simulink model "LAB_BalancingRobotSim"  (R2020b)
settings: Solver=FixedStepDiscrete  StartTime=0.0  StopTime=10.0  FixedStep=0.01  RelTol=1e-3  EnableMultiTasking=on
undefined symbols (not defined in the file): D_CF, DiscIntNeverNeededParam, drv, gbox, H, K, K_I, Ki_yaw, Kp_yaw, N_CF, Nu, Nx, psi_ref, sens, Ts, wheel
libraries: BalRobTbx_baselib x15
settings Model: SILPILModeSetting=veronly  ExtModeTrigDuration=2  Creator=barondavid  LastModifiedBy=Musta
settings OptimizationCC: EnhancedBackFolding=on  PassReuseOutputArgsAs=Individual arguments  ZeroExternalMemoryAtStartup=off  ZeroInternalMemoryAtStartup=off  MaxStackSize=64  OptimizeBlockOrder=speed  DifferentSizesBufferReuse=on  OptimizationCustomize=off  EfficientTunableParamExpr=on
settings DebuggingCC: ParameterTunabilityLossMsg=error
settings HardwareCC: ProdBitPerInt=16  ProdBitPerPointer=16  ProdBitPerSizeT=16  ProdBitPerPtrDiffT=16  ProdLargestAtomicFloat=None  ProdWordSize=8  ProdHWDeviceType=Atmel->AVR
settings SFSimCC: MATLABDynamicMemAlloc=off
settings RTWCC: Description=Embedded Coder  SystemTargetFile=ert.tlc  HardwareBoard=Arduino Mega 2560  TemplateMakefile=ert_default_tmf  Toolchain=Arduino AVR  BuildConfiguration=Faster Runs
settings CodeAppCC: ForceParamTrailComments=on  IgnoreCustomStorageClasses=off  OperatorAnnotations=on  SimulinkDataObjDesc=on  SFDataObjDesc=on  InsertBlockDesc=on
settings ERTTargetCC: SupportContinuousTime=on  SupportVariableSizeSignals=on  ExtModeStaticAllocSize=2048

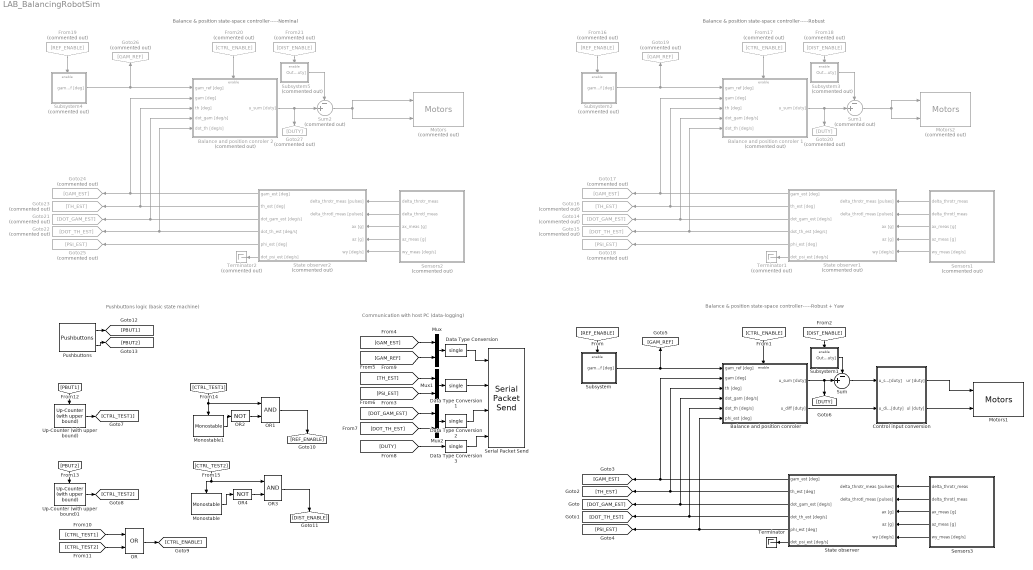
== system LAB_BalancingRobotSim ==
  note: Balance & position state-space controller-----Robust
  note: Pushbuttons logic (basic state machine)
  note: Balance & position state-space controller-----Robust + Yaw
  note: Communication with host PC (data-logging)
  note: Balance & position state-space controller-----Nominal
  "Balance and position conroler " : Subsystem
  Balance and position conroler 1 : Subsystem  Commented=on
  Balance and position conroler 2 : Subsystem  Commented=on
  Control input conversion : Subsystem
  Data Type Conversion{,1..3} (4 alike) : DataTypeConversion  OutDataTypeStr=single
  From16 : From  Commented=on  GotoTag=REF_ENABLE
  From17 : From  Commented=on  GotoTag=CTRL_ENABLE
  From18 : From  Commented=on  GotoTag=DIST_ENABLE
  From19 : From  Commented=on  GotoTag=REF_ENABLE
  From20 : From  Commented=on  GotoTag=CTRL_ENABLE
  From21 : From  Commented=on  GotoTag=DIST_ENABLE
  Goto14 : Goto  Commented=on  GotoTag=DOT_GAM_EST
  Goto15 : Goto  Commented=on  GotoTag=DOT_TH_EST
  Goto16 : Goto  Commented=on  GotoTag=TH_EST
  Goto17 : Goto  Commented=on  GotoTag=GAM_EST
  Goto18 : Goto  Commented=on  GotoTag=PSI_EST
  Goto19 : Goto  Commented=on  GotoTag=GAM_REF
  Goto20 : Goto  Commented=on  GotoTag=DUTY
  Goto21 : Goto  Commented=on  GotoTag=DOT_GAM_EST
  Goto22 : Goto  Commented=on  GotoTag=DOT_TH_EST
  Goto23 : Goto  Commented=on  GotoTag=TH_EST
  Goto24 : Goto  Commented=on  GotoTag=GAM_EST
  Goto25 : Goto  Commented=on  GotoTag=PSI_EST
  Goto26 : Goto  Commented=on  GotoTag=GAM_REF
  Goto27 : Goto  Commented=on  GotoTag=DUTY
  Monostable : BalRobTbx_baselib/Utilities/Monostable  Tp=20
      settings: SourceProductName=Balancing Robot Toolbox
  Monostable1 : BalRobTbx_baselib/Utilities/Monostable  Tp=10
      settings: SourceProductName=Balancing Robot Toolbox
  Motors : BalRobTbx_baselib/Outputs/Motors  Commented=on
      settings: SourceProductName=Balancing Robot Toolbox
  Motors1 : BalRobTbx_baselib/Outputs/Motors
      settings: SourceProductName=Balancing Robot Toolbox
  Motors2 : BalRobTbx_baselib/Outputs/Motors  Commented=on
      settings: SourceProductName=Balancing Robot Toolbox
  Mux : Mux  Inputs=2
  Mux1 : Mux  Inputs=2
  Mux2 : Mux  Inputs=2
  OR : Logic  Operator=OR  AllPortsSameDT=off  OutDataTypeStr=boolean
  OR1 : Logic  AllPortsSameDT=off  OutDataTypeStr=boolean
  OR2 : Logic  Operator=NOT  AllPortsSameDT=off  OutDataTypeStr=boolean
  OR3 : Logic  AllPortsSameDT=off  OutDataTypeStr=boolean
  OR4 : Logic  Operator=NOT  AllPortsSameDT=off  OutDataTypeStr=boolean
  Pushbuttons : BalRobTbx_baselib/Inputs/Pushbuttons
      settings: SourceProductName=Balancing Robot Toolbox
  Sensors1 : Subsystem  Commented=on
  Sensors2 : Subsystem  Commented=on
  Sensors3 : Subsystem
  Serial Packet Send : BalRobTbx_baselib/Communication/Serial Packet Send  serialLinkOpt=Bluetooth  baudRateOpt=38400  waitHostTxCmd=on  txStartCmd=65  txStopCmd=66  packetSpec={'2*single','2*single','2*single','1*single'}  cobsEncoded=on  nullTerminated=on  showEnablePort=off
      settings: SourceProductName=Balancing Robot Toolbox
  State observer : Subsystem
  State observer1 : Subsystem  Commented=on
  State observer2 : Subsystem  Commented=on
  Subsystem : Subsystem
  Subsystem1 : Subsystem
  Subsystem2 : Subsystem  Commented=on
  Subsystem3 : Subsystem  Commented=on
  Subsystem4 : Subsystem  Commented=on
  Subsystem5 : Subsystem  Commented=on
  Sum : Sum  Inputs=-+|
  Sum1 : Sum  Commented=on  Inputs=-+|
  Sum2 : Sum  Commented=on  Inputs=-+|
  Terminator : Terminator
  Terminator1 : Terminator  Commented=on
  Terminator2 : Terminator  Commented=on
  Up-Counter (with upper bound) : BalRobTbx_baselib/Utilities/Up-Counter (with upper bound)  CMAX=10  C0=0
      settings: SourceProductName=Balancing Robot Toolbox
  Up-Counter (with upper bound)1 : BalRobTbx_baselib/Utilities/Up-Counter (with upper bound)  CMAX=10  C0=0
      settings: SourceProductName=Balancing Robot Toolbox
  wires:
  Subsystem3/1(Out [duty]) -> Sum1/1
  Mux1/1 -> Data Type Conversion1/1
  Sensors3/3(ax_meas [g]) -> State observer/3(ax [g])
  [REF_ENABLE] -> Subsystem/Enable
  Sensors2/2(delta_throtl_meas) -> State observer2/2(delta_throtl_meas [pulses])
  [DIST_ENABLE] -> Subsystem1/Enable
  Mux/1 -> Data Type Conversion/1
  Mux2/1 -> Data Type Conversion2/1
  Sensors1/5(wy_meas [deg/s]) -> State observer1/5(wy [deg/s])
  State observer2/5(phi_est [deg]) -> Goto25/1
  "Balance and position conroler "/1(u_sum [duty]) -> [DUTY], Sum/2
  OR4/1 -> OR3/2
  Sensors2/1(delta_throtr_meas) -> State observer2/1(delta_throtr_meas [pulses])
  [GAM_REF] -> Mux/2
  [CTRL_ENABLE] -> "Balance and position conroler "/Enable
  Sensors2/4(az_meas [g]) -> State observer2/4(az [g])
  Subsystem2/1(gam_ref [deg]) -> Goto19/1, Balance and position conroler 1/1(gam_ref [deg])
  Subsystem4/1(gam_ref [deg]) -> Goto26/1, Balance and position conroler 2/1(gam_ref [deg])
  From19/1 -> Subsystem4/Enable
  [TH_EST] -> Mux1/1
  From21/1 -> Subsystem5/Enable
  OR/1 -> [CTRL_ENABLE]
  Sensors3/4(az_meas [g]) -> State observer/4(az [g])
  State observer1/1(gam_est [deg]) -> Goto17/1, Balance and position conroler 1/2(gam [deg])
  State observer2/6(dot_psi_est [deg/s]) -> Terminator2/1
  Sensors1/4(az_meas [g]) -> State observer1/4(az [g])
  Balance and position conroler 2/1(u_sum [duty]) -> Goto27/1, Sum2/2
  State observer2/3(dot_gam_est [deg/s]) -> Balance and position conroler 2/4(dot_gam [deg/s]), Goto21/1
  From16/1 -> Subsystem2/Enable
  [GAM_EST] -> Mux/1
  State observer/6(dot_psi_est [deg/s]) -> Terminator/1
  [CTRL_TEST1] -> Monostable1/Enable, OR1/1
  Subsystem1/1(Out [duty]) -> Sum/1
  State observer2/4(dot_th_est [deg/s]) -> Balance and position conroler 2/5(dot_th [deg/s]), Goto22/1
  From17/1 -> Balance and position conroler 1/Enable
  Sensors2/3(ax_meas [g]) -> State observer2/3(ax [g])
  State observer/2(th_est [deg]) -> [TH_EST], "Balance and position conroler "/3(th [deg])
  OR2/1 -> OR1/2
  State observer1/2(th_est [deg]) -> Goto16/1, Balance and position conroler 1/3(th [deg])
  Sensors2/5(wy_meas [deg/s]) -> State observer2/5(wy [deg/s])
  State observer1/5(phi_est [deg]) -> Goto18/1
  From18/1 -> Subsystem3/Enable
  [DOT_GAM_EST] -> Mux2/1
  Sum/1 -> Control input conversion/1(u_sum [duty])
  State observer1/3(dot_gam_est [deg/s]) -> Balance and position conroler 1/4(dot_gam [deg/s]), Goto14/1
  Subsystem5/1(Out [duty]) -> Sum2/1
  [CTRL_TEST2] -> Monostable/Enable, OR3/1
  Subsystem/1(gam_ref [deg]) -> "Balance and position conroler "/1(gam_ref [deg]), [GAM_REF]
  State observer1/6(dot_psi_est [deg/s]) -> Terminator1/1
  Sensors1/2(delta_throtl_meas) -> State observer1/2(delta_throtl_meas [pulses])
  State observer1/4(dot_th_est [deg/s]) -> Balance and position conroler 1/5(dot_th [deg/s]), Goto15/1
  [CTRL_TEST1] -> OR/1
  Sensors3/1(delta_throtr_meas) -> State observer/1(delta_throtr_meas [pulses])
  Sensors3/2(delta_throtl_meas) -> State observer/2(delta_throtl_meas [pulses])
  Sensors1/1(delta_throtr_meas) -> State observer1/1(delta_throtr_meas [pulses])
  [PSI_EST] -> Mux1/2
  State observer/5(phi_est [deg]) -> [PSI_EST], "Balance and position conroler "/6(phi_est [deg])
  State observer/4(dot_th_est [deg/s]) -> "Balance and position conroler "/5(dot_th [deg/s]), [DOT_TH_EST]
  From20/1 -> Balance and position conroler 2/Enable
  "Balance and position conroler "/2(u_diff [duty]) -> Control input conversion/2(u_diff [duty])
  Sensors3/5(wy_meas [deg/s]) -> State observer/5(wy [deg/s])
  [CTRL_TEST2] -> OR/2
  State observer2/1(gam_est [deg]) -> Goto24/1, Balance and position conroler 2/2(gam [deg])
  State observer/1(gam_est [deg]) -> [GAM_EST], "Balance and position conroler "/2(gam [deg])
  State observer2/2(th_est [deg]) -> Goto23/1, Balance and position conroler 2/3(th [deg])
  State observer/3(dot_gam_est [deg/s]) -> "Balance and position conroler "/4(dot_gam [deg/s]), [DOT_GAM_EST]
  Balance and position conroler 1/1(u_sum [duty]) -> Goto20/1, Sum1/2
  [DOT_TH_EST] -> Mux2/2
  Sensors1/3(ax_meas [g]) -> State observer1/3(ax [g])
  Pushbuttons/1 -> [PBUT1]
  Pushbuttons/2 -> [PBUT2]
  Up-Counter (with upper bound)/1 -> [CTRL_TEST1]
  Up-Counter (with upper bound)1/1 -> [CTRL_TEST2]
  Monostable1/1 -> OR2/1
  Monostable/1 -> OR4/1
  Data Type Conversion/1 -> Serial Packet Send/1
  Data Type Conversion1/1 -> Serial Packet Send/2
  Data Type Conversion2/1 -> Serial Packet Send/3
  Data Type Conversion3/1 -> Serial Packet Send/4
  [PBUT1] -> Up-Counter (with upper bound)/Trigger
  [PBUT2] -> Up-Counter (with upper bound)1/Trigger
  Sum2/1 -> Motors/2, Motors/1
  OR1/1 -> [REF_ENABLE]
  OR3/1 -> [DIST_ENABLE]
  [DUTY] -> Data Type Conversion3/1
  Control input conversion/1(ur [duty]) -> Motors1/1
  Control input conversion/2(ul [duty]) -> Motors1/2
  Sum1/1 -> Motors2/1, Motors2/2

== system LAB_BalancingRobotSim/Balance and position conroler  ==
  gam_ref [deg] : Inport
  gam [deg] : Inport  Port=2
  th [deg] : Inport  Port=3
  dot_gam [deg/s] : Inport  Port=4
  dot_th [deg/s] : Inport  Port=5
  phi_est [deg] : Inport  Port=6
  Enable : EnablePort
  Lateral (Yaw) controller : Subsystem
  Longitudinal controller : Subsystem
  u_sum [duty] : Outport
  u_diff [duty] : Outport  Port=2
  wires:
  dot_gam [deg/s]/1 -> Longitudinal controller/4(dot_gam [deg/s])
  gam_ref [deg]/1 -> Longitudinal controller/1(gam_ref [deg])
  Longitudinal controller/1(u [duty]) -> u_sum [duty]/1
  th [deg]/1 -> Longitudinal controller/3(th [deg])
  phi_est [deg]/1 -> Lateral (Yaw) controller/1(phi_est [deg])
  gam [deg]/1 -> Longitudinal controller/2(gam [deg])
  dot_th [deg/s]/1 -> Longitudinal controller/5(dot_th [deg/s])
  Lateral (Yaw) controller/1(u_diff [duty]) -> u_diff [duty]/1

== system LAB_BalancingRobotSim/Balance and position conroler 1 ==
  gam_ref [deg] : Inport
  gam [deg] : Inport  Port=2
  th [deg] : Inport  Port=3
  dot_gam [deg/s] : Inport  Port=4
  dot_th [deg/s] : Inport  Port=5
  Enable : EnablePort
  Longitudinal controller : Subsystem
  u_sum [duty] : Outport
  wires:
  dot_gam [deg/s]/1 -> Longitudinal controller/4(dot_gam [deg/s])
  gam_ref [deg]/1 -> Longitudinal controller/1(gam_ref [deg])
  Longitudinal controller/1(u [duty]) -> u_sum [duty]/1
  th [deg]/1 -> Longitudinal controller/3(th [deg])
  gam [deg]/1 -> Longitudinal controller/2(gam [deg])
  dot_th [deg/s]/1 -> Longitudinal controller/5(dot_th [deg/s])

== system LAB_BalancingRobotSim/Balance and position conroler 2 ==
  gam_ref [deg] : Inport
  gam [deg] : Inport  Port=2
  th [deg] : Inport  Port=3
  dot_gam [deg/s] : Inport  Port=4
  dot_th [deg/s] : Inport  Port=5
  Enable : EnablePort
  Longitudinal controller : Subsystem
  u_sum [duty] : Outport
  wires:
  dot_gam [deg/s]/1 -> Longitudinal controller/4(dot_gam [deg/s])
  gam_ref [deg]/1 -> Longitudinal controller/1(gam_ref [deg])
  Longitudinal controller/1(u [duty]) -> u_sum [duty]/1
  th [deg]/1 -> Longitudinal controller/3(th [deg])
  gam [deg]/1 -> Longitudinal controller/2(gam [deg])
  dot_th [deg/s]/1 -> Longitudinal controller/5(dot_th [deg/s])

== system LAB_BalancingRobotSim/Control input conversion ==
  u_sum [duty] : Inport
  u_diff [duty] : Inport  Port=2
  Sum1 : Sum
  Sum3 : Sum  Inputs=+-
  ur [duty] : Outport
  ul [duty] : Outport  Port=2
  wires:
  u_diff [duty]/1 -> Sum1/2, Sum3/2
  Sum1/1 -> ur [duty]/1
  Sum3/1 -> ul [duty]/1
  u_sum [duty]/1 -> Sum3/1, Sum1/1

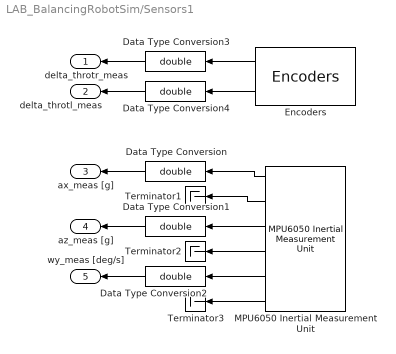
== system LAB_BalancingRobotSim/Sensors1 ==
  Data Type Conversion{,1..4} (5 alike) : DataTypeConversion  OutDataTypeStr=double
  Encoders : BalRobTbx_baselib/Inputs/Encoders
      settings: SourceProductName=Balancing Robot Toolbox
  MPU6050 Inertial Measurement Unit : BalRobTbx_baselib/Inputs/MPU6050 Inertial Measurement Unit
      settings: SourceProductName=Balancing Robot Toolbox
  Terminator1 : Terminator
  Terminator2 : Terminator
  Terminator3 : Terminator
  delta_throtr_meas : Outport
  delta_throtl_meas : Outport  Port=2
  ax_meas [g] : Outport  Port=3
  az_meas [g] : Outport  Port=4
  wy_meas [deg/s] : Outport  Port=5
  wires:
  Data Type Conversion1/1 -> az_meas [g]/1
  Data Type Conversion/1 -> ax_meas [g]/1
  Data Type Conversion2/1 -> wy_meas [deg/s]/1
  Data Type Conversion4/1 -> delta_throtl_meas/1
  Data Type Conversion3/1 -> delta_throtr_meas/1
  Encoders/1 -> Data Type Conversion3/1
  MPU6050 Inertial Measurement Unit/5 -> Data Type Conversion2/1
  MPU6050 Inertial Measurement Unit/6 -> Terminator3/1
  MPU6050 Inertial Measurement Unit/4 -> Terminator2/1
  Encoders/2 -> Data Type Conversion4/1
  MPU6050 Inertial Measurement Unit/1 -> Data Type Conversion/1
  MPU6050 Inertial Measurement Unit/3 -> Data Type Conversion1/1
  MPU6050 Inertial Measurement Unit/2 -> Terminator1/1

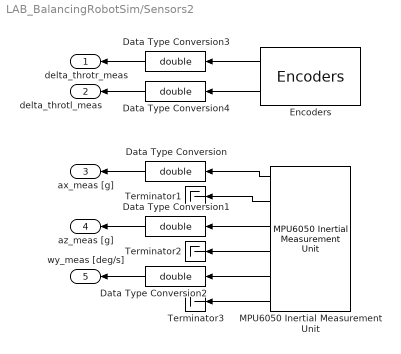
== system LAB_BalancingRobotSim/Sensors2 ==
  Data Type Conversion{,1..4} (5 alike) : DataTypeConversion  OutDataTypeStr=double
  Encoders : BalRobTbx_baselib/Inputs/Encoders
      settings: SourceProductName=Balancing Robot Toolbox
  MPU6050 Inertial Measurement Unit : BalRobTbx_baselib/Inputs/MPU6050 Inertial Measurement Unit
      settings: SourceProductName=Balancing Robot Toolbox
  Terminator1 : Terminator
  Terminator2 : Terminator
  Terminator3 : Terminator
  delta_throtr_meas : Outport
  delta_throtl_meas : Outport  Port=2
  ax_meas [g] : Outport  Port=3
  az_meas [g] : Outport  Port=4
  wy_meas [deg/s] : Outport  Port=5
  wires:
  Data Type Conversion1/1 -> az_meas [g]/1
  Data Type Conversion/1 -> ax_meas [g]/1
  Data Type Conversion2/1 -> wy_meas [deg/s]/1
  Data Type Conversion4/1 -> delta_throtl_meas/1
  Data Type Conversion3/1 -> delta_throtr_meas/1
  Encoders/1 -> Data Type Conversion3/1
  Encoders/2 -> Data Type Conversion4/1
  MPU6050 Inertial Measurement Unit/1 -> Data Type Conversion/1
  MPU6050 Inertial Measurement Unit/2 -> Terminator1/1
  MPU6050 Inertial Measurement Unit/3 -> Data Type Conversion1/1
  MPU6050 Inertial Measurement Unit/4 -> Terminator2/1
  MPU6050 Inertial Measurement Unit/5 -> Data Type Conversion2/1
  MPU6050 Inertial Measurement Unit/6 -> Terminator3/1

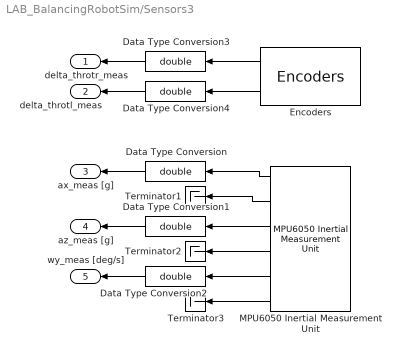
== system LAB_BalancingRobotSim/Sensors3 ==
  Data Type Conversion{,1..4} (5 alike) : DataTypeConversion  OutDataTypeStr=double
  Encoders : BalRobTbx_baselib/Inputs/Encoders
      settings: SourceProductName=Balancing Robot Toolbox
  MPU6050 Inertial Measurement Unit : BalRobTbx_baselib/Inputs/MPU6050 Inertial Measurement Unit
      settings: SourceProductName=Balancing Robot Toolbox
  Terminator1 : Terminator
  Terminator2 : Terminator
  Terminator3 : Terminator
  delta_throtr_meas : Outport
  delta_throtl_meas : Outport  Port=2
  ax_meas [g] : Outport  Port=3
  az_meas [g] : Outport  Port=4
  wy_meas [deg/s] : Outport  Port=5
  wires:
  MPU6050 Inertial Measurement Unit/6 -> Terminator3/1
  MPU6050 Inertial Measurement Unit/5 -> Data Type Conversion2/1
  MPU6050 Inertial Measurement Unit/4 -> Terminator2/1
  MPU6050 Inertial Measurement Unit/3 -> Data Type Conversion1/1
  MPU6050 Inertial Measurement Unit/2 -> Terminator1/1
  MPU6050 Inertial Measurement Unit/1 -> Data Type Conversion/1
  Encoders/2 -> Data Type Conversion4/1
  Encoders/1 -> Data Type Conversion3/1
  Data Type Conversion3/1 -> delta_throtr_meas/1
  Data Type Conversion4/1 -> delta_throtl_meas/1
  Data Type Conversion2/1 -> wy_meas [deg/s]/1
  Data Type Conversion/1 -> ax_meas [g]/1
  Data Type Conversion1/1 -> az_meas [g]/1

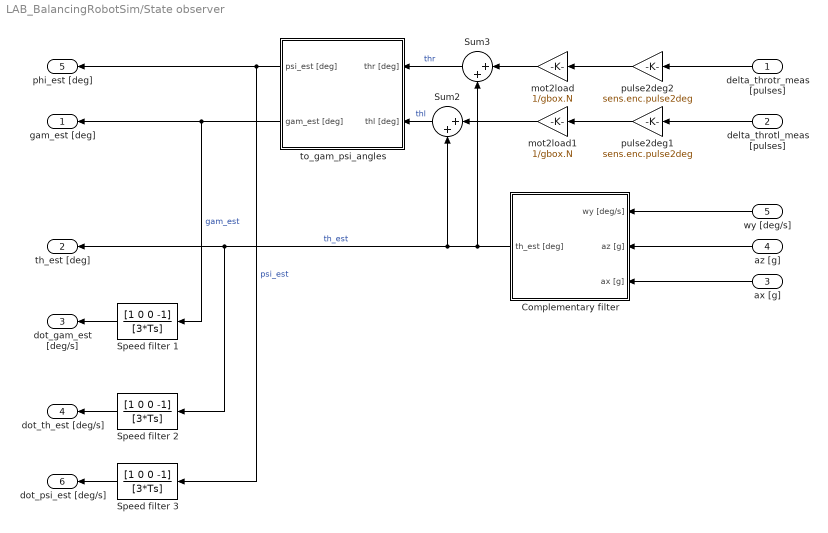
== system LAB_BalancingRobotSim/State observer ==
  delta_throtr_meas [pulses] : Inport
  delta_throtl_meas [pulses] : Inport  Port=2
  ax [g] : Inport  Port=3
  az [g] : Inport  Port=4
  wy [deg/s] : Inport  Port=5
  Complementary filter : Subsystem
  Speed filter 1 : DiscreteFilter  Numerator=[1 0 0 -1]  Denominator=[3*Ts]  SampleTime=Ts
  Speed filter 2 : DiscreteFilter  Numerator=[1 0 0 -1]  Denominator=[3*Ts]  SampleTime=Ts
  Speed filter 3 : DiscreteFilter  Numerator=[1 0 0 -1]  Denominator=[3*Ts]  SampleTime=Ts
  Sum2 : Sum  Inputs=|++
  Sum3 : Sum  Inputs=|++
  mot2load : Gain  Gain=1/gbox.N
  mot2load1 : Gain  Gain=1/gbox.N
  pulse2deg1 : Gain  Gain=sens.enc.pulse2deg
  pulse2deg2 : Gain  Gain=sens.enc.pulse2deg
  to_gam_psi_angles : Subsystem
  gam_est [deg] : Outport
  th_est [deg] : Outport  Port=2
  dot_gam_est [deg/s] : Outport  Port=3
  dot_th_est [deg/s] : Outport  Port=4
  phi_est [deg] : Outport  Port=5
  dot_psi_est [deg/s] : Outport  Port=6
  wires:
  Speed filter 2/1 -> dot_th_est [deg/s]/1
  ax [g]/1 -> Complementary filter/3(ax [g])
  az [g]/1 -> Complementary filter/2(az [g])
  wy [deg/s]/1 -> Complementary filter/1(wy [deg/s])
  Speed filter 1/1 -> dot_gam_est [deg/s]/1
  delta_throtl_meas [pulses]/1 -> pulse2deg1/1
  mot2load1/1 -> Sum2/1
  mot2load/1 -> Sum3/1
  delta_throtr_meas [pulses]/1 -> pulse2deg2/1
  Complementary filter/1(th_est [deg]) -> th_est [deg]/1, Speed filter 2/1, Sum2/2, Sum3/2  "th_est"
  pulse2deg1/1 -> mot2load1/1
  pulse2deg2/1 -> mot2load/1
  Sum3/1 -> to_gam_psi_angles/1(thr [deg])  "thr"
  Sum2/1 -> to_gam_psi_angles/2(thl [deg])  "thl"
  to_gam_psi_angles/1(psi_est [deg]) -> Speed filter 3/1, phi_est [deg]/1  "psi_est"
  to_gam_psi_angles/2(gam_est [deg]) -> gam_est [deg]/1, Speed filter 1/1  "gam_est"
  Speed filter 3/1 -> dot_psi_est [deg/s]/1

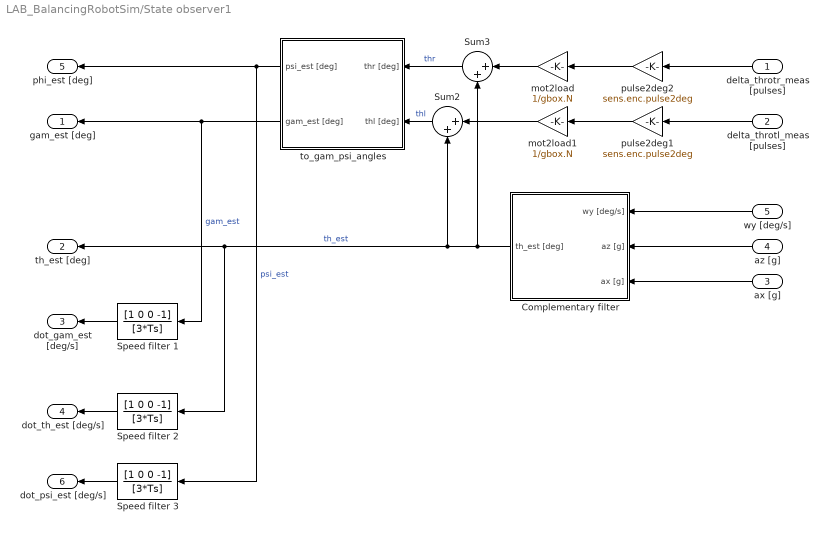
== system LAB_BalancingRobotSim/State observer1 ==
  delta_throtr_meas [pulses] : Inport
  delta_throtl_meas [pulses] : Inport  Port=2
  ax [g] : Inport  Port=3
  az [g] : Inport  Port=4
  wy [deg/s] : Inport  Port=5
  Complementary filter : Subsystem
  Speed filter 1 : DiscreteFilter  Numerator=[1 0 0 -1]  Denominator=[3*Ts]  SampleTime=Ts
  Speed filter 2 : DiscreteFilter  Numerator=[1 0 0 -1]  Denominator=[3*Ts]  SampleTime=Ts
  Speed filter 3 : DiscreteFilter  Numerator=[1 0 0 -1]  Denominator=[3*Ts]  SampleTime=Ts
  Sum2 : Sum  Inputs=|++
  Sum3 : Sum  Inputs=|++
  mot2load : Gain  Gain=1/gbox.N
  mot2load1 : Gain  Gain=1/gbox.N
  pulse2deg1 : Gain  Gain=sens.enc.pulse2deg
  pulse2deg2 : Gain  Gain=sens.enc.pulse2deg
  to_gam_psi_angles : Subsystem
  gam_est [deg] : Outport
  th_est [deg] : Outport  Port=2
  dot_gam_est [deg/s] : Outport  Port=3
  dot_th_est [deg/s] : Outport  Port=4
  phi_est [deg] : Outport  Port=5
  dot_psi_est [deg/s] : Outport  Port=6
  wires:
  Speed filter 2/1 -> dot_th_est [deg/s]/1
  ax [g]/1 -> Complementary filter/3(ax [g])
  az [g]/1 -> Complementary filter/2(az [g])
  wy [deg/s]/1 -> Complementary filter/1(wy [deg/s])
  Speed filter 1/1 -> dot_gam_est [deg/s]/1
  delta_throtl_meas [pulses]/1 -> pulse2deg1/1
  mot2load1/1 -> Sum2/1
  mot2load/1 -> Sum3/1
  delta_throtr_meas [pulses]/1 -> pulse2deg2/1
  Complementary filter/1(th_est [deg]) -> th_est [deg]/1, Speed filter 2/1, Sum2/2, Sum3/2  "th_est"
  pulse2deg1/1 -> mot2load1/1
  pulse2deg2/1 -> mot2load/1
  Sum3/1 -> to_gam_psi_angles/1(thr [deg])  "thr"
  Sum2/1 -> to_gam_psi_angles/2(thl [deg])  "thl"
  to_gam_psi_angles/1(psi_est [deg]) -> Speed filter 3/1, phi_est [deg]/1  "psi_est"
  to_gam_psi_angles/2(gam_est [deg]) -> gam_est [deg]/1, Speed filter 1/1  "gam_est"
  Speed filter 3/1 -> dot_psi_est [deg/s]/1

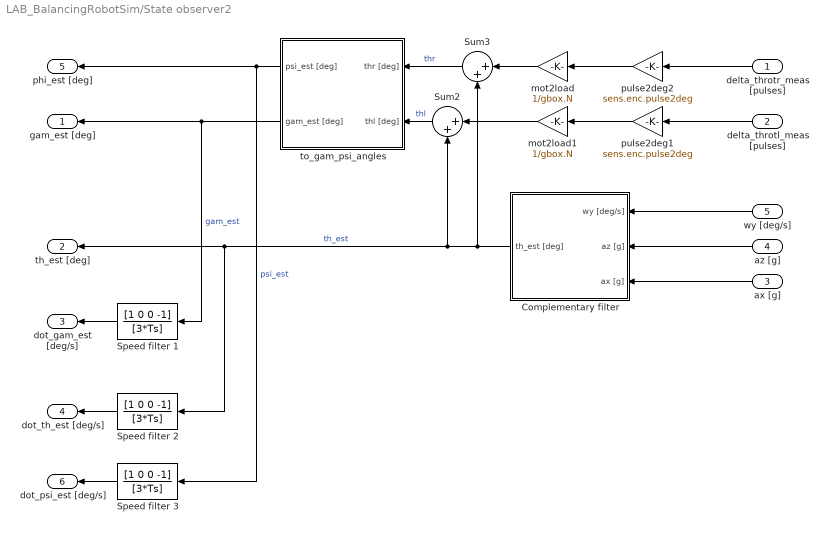
== system LAB_BalancingRobotSim/State observer2 ==
  delta_throtr_meas [pulses] : Inport
  delta_throtl_meas [pulses] : Inport  Port=2
  ax [g] : Inport  Port=3
  az [g] : Inport  Port=4
  wy [deg/s] : Inport  Port=5
  Complementary filter : Subsystem
  Speed filter 1 : DiscreteFilter  Numerator=[1 0 0 -1]  Denominator=[3*Ts]  SampleTime=Ts
  Speed filter 2 : DiscreteFilter  Numerator=[1 0 0 -1]  Denominator=[3*Ts]  SampleTime=Ts
  Speed filter 3 : DiscreteFilter  Numerator=[1 0 0 -1]  Denominator=[3*Ts]  SampleTime=Ts
  Sum2 : Sum  Inputs=|++
  Sum3 : Sum  Inputs=|++
  mot2load : Gain  Gain=1/gbox.N
  mot2load1 : Gain  Gain=1/gbox.N
  pulse2deg1 : Gain  Gain=sens.enc.pulse2deg
  pulse2deg2 : Gain  Gain=sens.enc.pulse2deg
  to_gam_psi_angles : Subsystem
  gam_est [deg] : Outport
  th_est [deg] : Outport  Port=2
  dot_gam_est [deg/s] : Outport  Port=3
  dot_th_est [deg/s] : Outport  Port=4
  phi_est [deg] : Outport  Port=5
  dot_psi_est [deg/s] : Outport  Port=6
  wires:
  Speed filter 2/1 -> dot_th_est [deg/s]/1
  ax [g]/1 -> Complementary filter/3(ax [g])
  az [g]/1 -> Complementary filter/2(az [g])
  wy [deg/s]/1 -> Complementary filter/1(wy [deg/s])
  Speed filter 1/1 -> dot_gam_est [deg/s]/1
  delta_throtl_meas [pulses]/1 -> pulse2deg1/1
  mot2load1/1 -> Sum2/1
  mot2load/1 -> Sum3/1
  delta_throtr_meas [pulses]/1 -> pulse2deg2/1
  Complementary filter/1(th_est [deg]) -> th_est [deg]/1, Speed filter 2/1, Sum2/2, Sum3/2  "th_est"
  pulse2deg1/1 -> mot2load1/1
  pulse2deg2/1 -> mot2load/1
  Sum3/1 -> to_gam_psi_angles/1(thr [deg])  "thr"
  Sum2/1 -> to_gam_psi_angles/2(thl [deg])  "thl"
  to_gam_psi_angles/1(psi_est [deg]) -> Speed filter 3/1, phi_est [deg]/1  "psi_est"
  to_gam_psi_angles/2(gam_est [deg]) -> gam_est [deg]/1, Speed filter 1/1  "gam_est"
  Speed filter 3/1 -> dot_psi_est [deg/s]/1

== system LAB_BalancingRobotSim/Subsystem ==
  Enable : EnablePort
  Zero : Constant  Value=(2*0.1/wheel.r)*rad2deg  OutDataTypeStr=Inherit: Inherit via back propagation
  gam_ref [deg] : Outport  OutputWhenDisabled=reset  InitialOutput=0
  wires:
  Zero/1 -> gam_ref [deg]/1

== system LAB_BalancingRobotSim/Subsystem1 ==
  Enable : EnablePort
  Zero : Constant  Value=5.0/drv.duty2V  OutDataTypeStr=Inherit: Inherit via back propagation
  Out [duty] : Outport  OutputWhenDisabled=reset  InitialOutput=0
  wires:
  Zero/1 -> Out [duty]/1

== system LAB_BalancingRobotSim/Subsystem2 ==
  Enable : EnablePort
  Zero : Constant  Value=(0.1/wheel.r)*rad2deg  OutDataTypeStr=Inherit: Inherit via back propagation
  gam_ref [deg] : Outport  OutputWhenDisabled=reset  InitialOutput=0
  wires:
  Zero/1 -> gam_ref [deg]/1

== system LAB_BalancingRobotSim/Subsystem3 ==
  Enable : EnablePort
  Zero : Constant  Value=5.0/drv.duty2V  OutDataTypeStr=Inherit: Inherit via back propagation
  Out [duty] : Outport  OutputWhenDisabled=reset  InitialOutput=0
  wires:
  Zero/1 -> Out [duty]/1

== system LAB_BalancingRobotSim/Subsystem4 ==
  Enable : EnablePort
  Zero : Constant  Value=(0.1/wheel.r)*rad2deg  OutDataTypeStr=Inherit: Inherit via back propagation
  gam_ref [deg] : Outport  OutputWhenDisabled=reset  InitialOutput=0
  wires:
  Zero/1 -> gam_ref [deg]/1

== system LAB_BalancingRobotSim/Subsystem5 ==
  Enable : EnablePort
  Zero : Constant  Value=5.0/drv.duty2V  OutDataTypeStr=Inherit: Inherit via back propagation
  Out [duty] : Outport  OutputWhenDisabled=reset  InitialOutput=0
  wires:
  Zero/1 -> Out [duty]/1

== system LAB_BalancingRobotSim/Balance and position conroler /Lateral (Yaw) controller ==
  phi_est [deg] : Inport
  Discrete-Time Integrator : DiscreteIntegrator  SampleTime=Ts  ICPrevOutput=DiscIntNeverNeededParam  ICPrevScaledInput=DiscIntNeverNeededParam
  Integral gain : Gain  Gain=Ki_yaw
  Proportional gain : Gain  Gain=Kp_yaw
  Sum1 : Sum  Inputs=+|+
  Sum2 : Sum  Inputs=+-|
  V2duty : Gain  Gain=drv.V2duty
  Yaw angle reference : Step  Time=0  After=psi_ref  SampleTime=Ts
  deg2rad : Gain  Gain=deg2rad
  u_diff [duty] : Outport
  wires:
  Sum1/1 -> V2duty/1
  Proportional gain/1 -> Sum1/1
  deg2rad/1 -> Proportional gain/1, Integral gain/1  "error_yaw"
  Yaw angle reference/1 -> Sum2/1
  Sum2/1 -> deg2rad/1
  Integral gain/1 -> Discrete-Time Integrator/1
  Discrete-Time Integrator/1 -> Sum1/2
  phi_est [deg]/1 -> Sum2/2
  V2duty/1 -> u_diff [duty]/1

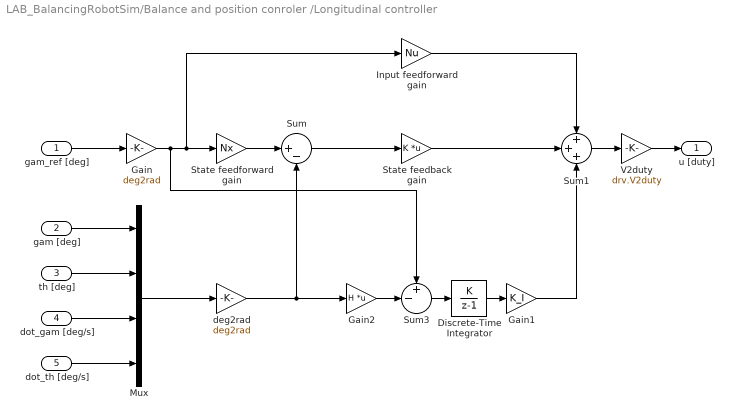
== system LAB_BalancingRobotSim/Balance and position conroler /Longitudinal controller ==
  gam_ref [deg] : Inport
  gam [deg] : Inport  Port=2
  th [deg] : Inport  Port=3
  dot_gam [deg/s] : Inport  Port=4
  dot_th [deg/s] : Inport  Port=5
  Discrete-Time Integrator : DiscreteIntegrator  IntegratorMethod=Accumulation: Forward Euler  SampleTime=Ts  ICPrevOutput=DiscIntNeverNeededParam  ICPrevScaledInput=DiscIntNeverNeededParam
  Gain : Gain  Gain=deg2rad
  Gain1 : Gain  Gain=K_I
  Gain2 : Gain  Gain=H  Multiplication=Matrix(K*u)
  Input feedforward gain : Gain  Gain=Nu
  Mux : Mux
  State feedback gain : Gain  Gain=K  Multiplication=Matrix(K*u)
  State feedforward gain : Gain  Gain=Nx
  Sum : Sum  Inputs=|+-
  Sum1 : Sum  Inputs=+++
  Sum3 : Sum  Inputs=+-|
  V2duty : Gain  Gain=drv.V2duty
  deg2rad : Gain  Gain=deg2rad
  u [duty] : Outport
  wires:
  gam [deg]/1 -> Mux/1
  th [deg]/1 -> Mux/2
  dot_gam [deg/s]/1 -> Mux/3
  dot_th [deg/s]/1 -> Mux/4
  Mux/1 -> deg2rad/1
  deg2rad/1 -> Gain2/1, Sum/2
  Sum/1 -> State feedback gain/1
  State feedback gain/1 -> Sum1/2
  Sum1/1 -> V2duty/1
  gam_ref [deg]/1 -> Gain/1
  State feedforward gain/1 -> Sum/1
  Input feedforward gain/1 -> Sum1/1
  Gain/1 -> Input feedforward gain/1, State feedforward gain/1, Sum3/1
  V2duty/1 -> u [duty]/1
  Sum3/1 -> Discrete-Time Integrator/1
  Discrete-Time Integrator/1 -> Gain1/1
  Gain1/1 -> Sum1/3
  Gain2/1 -> Sum3/2

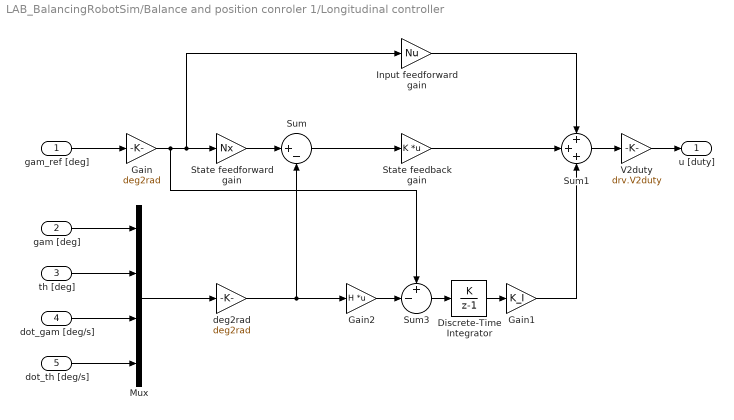
== system LAB_BalancingRobotSim/Balance and position conroler 1/Longitudinal controller ==
  gam_ref [deg] : Inport
  gam [deg] : Inport  Port=2
  th [deg] : Inport  Port=3
  dot_gam [deg/s] : Inport  Port=4
  dot_th [deg/s] : Inport  Port=5
  Discrete-Time Integrator : DiscreteIntegrator  IntegratorMethod=Accumulation: Forward Euler  SampleTime=Ts  ICPrevOutput=DiscIntNeverNeededParam  ICPrevScaledInput=DiscIntNeverNeededParam
  Gain : Gain  Gain=deg2rad
  Gain1 : Gain  Gain=K_I
  Gain2 : Gain  Gain=H  Multiplication=Matrix(K*u)
  Input feedforward gain : Gain  Gain=Nu
  Mux : Mux
  State feedback gain : Gain  Gain=K  Multiplication=Matrix(K*u)
  State feedforward gain : Gain  Gain=Nx
  Sum : Sum  Inputs=|+-
  Sum1 : Sum  Inputs=+++
  Sum3 : Sum  Inputs=+-|
  V2duty : Gain  Gain=drv.V2duty
  deg2rad : Gain  Gain=deg2rad
  u [duty] : Outport
  wires:
  gam [deg]/1 -> Mux/1
  th [deg]/1 -> Mux/2
  dot_gam [deg/s]/1 -> Mux/3
  dot_th [deg/s]/1 -> Mux/4
  Mux/1 -> deg2rad/1
  deg2rad/1 -> Gain2/1, Sum/2
  Sum/1 -> State feedback gain/1
  State feedback gain/1 -> Sum1/2
  Sum1/1 -> V2duty/1
  gam_ref [deg]/1 -> Gain/1
  State feedforward gain/1 -> Sum/1
  Input feedforward gain/1 -> Sum1/1
  Gain/1 -> Input feedforward gain/1, State feedforward gain/1, Sum3/1
  V2duty/1 -> u [duty]/1
  Sum3/1 -> Discrete-Time Integrator/1
  Discrete-Time Integrator/1 -> Gain1/1
  Gain1/1 -> Sum1/3
  Gain2/1 -> Sum3/2

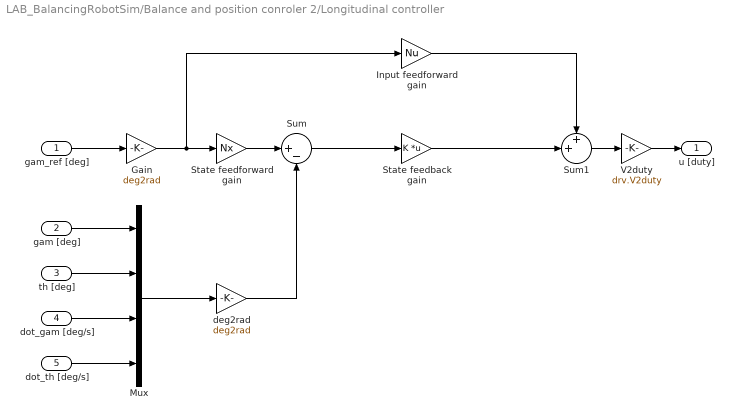
== system LAB_BalancingRobotSim/Balance and position conroler 2/Longitudinal controller ==
  gam_ref [deg] : Inport
  gam [deg] : Inport  Port=2
  th [deg] : Inport  Port=3
  dot_gam [deg/s] : Inport  Port=4
  dot_th [deg/s] : Inport  Port=5
  Gain : Gain  Gain=deg2rad
  Input feedforward gain : Gain  Gain=Nu
  Mux : Mux
  State feedback gain : Gain  Gain=K  Multiplication=Matrix(K*u)
  State feedforward gain : Gain  Gain=Nx
  Sum : Sum  Inputs=|+-
  Sum1 : Sum  Inputs=++|
  V2duty : Gain  Gain=drv.V2duty
  deg2rad : Gain  Gain=deg2rad
  u [duty] : Outport
  wires:
  gam [deg]/1 -> Mux/1
  th [deg]/1 -> Mux/2
  dot_gam [deg/s]/1 -> Mux/3
  dot_th [deg/s]/1 -> Mux/4
  Mux/1 -> deg2rad/1
  deg2rad/1 -> Sum/2
  Sum/1 -> State feedback gain/1
  State feedback gain/1 -> Sum1/2
  Sum1/1 -> V2duty/1
  gam_ref [deg]/1 -> Gain/1
  State feedforward gain/1 -> Sum/1
  Input feedforward gain/1 -> Sum1/1
  Gain/1 -> Input feedforward gain/1, State feedforward gain/1
  V2duty/1 -> u [duty]/1

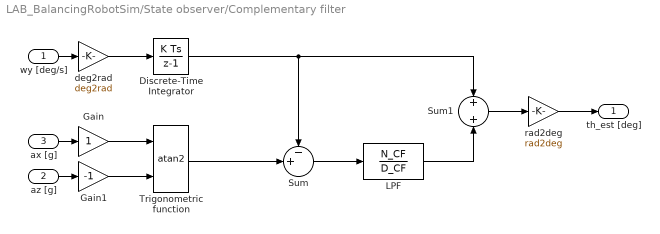
== system LAB_BalancingRobotSim/State observer/Complementary filter ==
  wy [deg/s] : Inport
  az [g] : Inport  Port=2
  ax [g] : Inport  Port=3
  Discrete-Time Integrator : DiscreteIntegrator  SampleTime=-1  ICPrevOutput=DiscIntNeverNeededParam  ICPrevScaledInput=DiscIntNeverNeededParam
  Gain : Gain
  Gain1 : Gain  Gain=-1
  LPF : DiscreteTransferFcn  Numerator=N_CF  Denominator=D_CF
  Sum : Sum  Inputs=-+|
  Sum1 : Sum  Inputs=+|+
  Trigonometric function : Trigonometry  Operator=atan2
  deg2rad : Gain  Gain=deg2rad
  rad2deg : Gain  Gain=rad2deg
  th_est [deg] : Outport
  wires:
  Discrete-Time Integrator/1 -> Sum1/1, Sum/1
  Gain1/1 -> Trigonometric function/2
  ax [g]/1 -> Gain/1
  Sum1/1 -> rad2deg/1
  Sum/1 -> LPF/1
  LPF/1 -> Sum1/2
  deg2rad/1 -> Discrete-Time Integrator/1
  Gain/1 -> Trigonometric function/1
  az [g]/1 -> Gain1/1
  rad2deg/1 -> th_est [deg]/1
  wy [deg/s]/1 -> deg2rad/1
  Trigonometric function/1 -> Sum/2

== system LAB_BalancingRobotSim/State observer/to_gam_psi_angles ==
  thr [deg] : Inport
  thl [deg] : Inport  Port=2
  Gain1 : Gain  Gain=0.5
  Gain3 : Gain  Gain=wheel.r/(2*wheel.yb)
  Sum1 : Sum  Inputs=++|
  Sum4 : Sum  Inputs=+-|
  psi_est [deg] : Outport
  gam_est [deg] : Outport  Port=2
  wires:
  thl [deg]/1 -> Sum1/2, Sum4/2
  Sum4/1 -> Gain3/1
  Gain3/1 -> psi_est [deg]/1
  thr [deg]/1 -> Sum1/1, Sum4/1
  Gain1/1 -> gam_est [deg]/1
  Sum1/1 -> Gain1/1

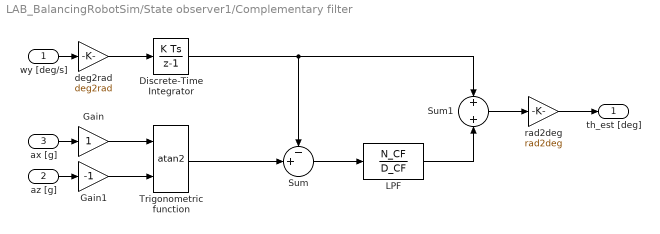
== system LAB_BalancingRobotSim/State observer1/Complementary filter ==
  wy [deg/s] : Inport
  az [g] : Inport  Port=2
  ax [g] : Inport  Port=3
  Discrete-Time Integrator : DiscreteIntegrator  SampleTime=-1  ICPrevOutput=DiscIntNeverNeededParam  ICPrevScaledInput=DiscIntNeverNeededParam
  Gain : Gain
  Gain1 : Gain  Gain=-1
  LPF : DiscreteTransferFcn  Numerator=N_CF  Denominator=D_CF
  Sum : Sum  Inputs=-+|
  Sum1 : Sum  Inputs=+|+
  Trigonometric function : Trigonometry  Operator=atan2
  deg2rad : Gain  Gain=deg2rad
  rad2deg : Gain  Gain=rad2deg
  th_est [deg] : Outport
  wires:
  Discrete-Time Integrator/1 -> Sum1/1, Sum/1
  Gain1/1 -> Trigonometric function/2
  ax [g]/1 -> Gain/1
  Sum1/1 -> rad2deg/1
  Sum/1 -> LPF/1
  LPF/1 -> Sum1/2
  deg2rad/1 -> Discrete-Time Integrator/1
  Gain/1 -> Trigonometric function/1
  az [g]/1 -> Gain1/1
  rad2deg/1 -> th_est [deg]/1
  wy [deg/s]/1 -> deg2rad/1
  Trigonometric function/1 -> Sum/2

== system LAB_BalancingRobotSim/State observer1/to_gam_psi_angles ==
  thr [deg] : Inport
  thl [deg] : Inport  Port=2
  Gain1 : Gain  Gain=0.5
  Gain3 : Gain  Gain=wheel.r/(2*wheel.yb)
  Sum1 : Sum  Inputs=++|
  Sum4 : Sum  Inputs=+-|
  psi_est [deg] : Outport
  gam_est [deg] : Outport  Port=2
  wires:
  thl [deg]/1 -> Sum1/2, Sum4/2
  Sum4/1 -> Gain3/1
  Gain3/1 -> psi_est [deg]/1
  thr [deg]/1 -> Sum1/1, Sum4/1
  Gain1/1 -> gam_est [deg]/1
  Sum1/1 -> Gain1/1

== system LAB_BalancingRobotSim/State observer2/Complementary filter ==
  wy [deg/s] : Inport
  az [g] : Inport  Port=2
  ax [g] : Inport  Port=3
  Discrete-Time Integrator : DiscreteIntegrator  SampleTime=-1  ICPrevOutput=DiscIntNeverNeededParam  ICPrevScaledInput=DiscIntNeverNeededParam
  Gain : Gain
  Gain1 : Gain  Gain=-1
  LPF : DiscreteTransferFcn  Numerator=N_CF  Denominator=D_CF
  Sum : Sum  Inputs=-+|
  Sum1 : Sum  Inputs=+|+
  Trigonometric function : Trigonometry  Operator=atan2
  deg2rad : Gain  Gain=deg2rad
  rad2deg : Gain  Gain=rad2deg
  th_est [deg] : Outport
  wires:
  Discrete-Time Integrator/1 -> Sum1/1, Sum/1
  Gain1/1 -> Trigonometric function/2
  ax [g]/1 -> Gain/1
  Sum1/1 -> rad2deg/1
  Sum/1 -> LPF/1
  LPF/1 -> Sum1/2
  deg2rad/1 -> Discrete-Time Integrator/1
  Gain/1 -> Trigonometric function/1
  az [g]/1 -> Gain1/1
  rad2deg/1 -> th_est [deg]/1
  wy [deg/s]/1 -> deg2rad/1
  Trigonometric function/1 -> Sum/2

== system LAB_BalancingRobotSim/State observer2/to_gam_psi_angles ==
  thr [deg] : Inport
  thl [deg] : Inport  Port=2
  Gain1 : Gain  Gain=0.5
  Gain3 : Gain  Gain=wheel.r/(2*wheel.yb)
  Sum1 : Sum  Inputs=++|
  Sum4 : Sum  Inputs=+-|
  psi_est [deg] : Outport
  gam_est [deg] : Outport  Port=2
  wires:
  thl [deg]/1 -> Sum1/2, Sum4/2
  Sum4/1 -> Gain3/1
  Gain3/1 -> psi_est [deg]/1
  thr [deg]/1 -> Sum1/1, Sum4/1
  Gain1/1 -> gam_est [deg]/1
  Sum1/1 -> Gain1/1
